simulink model "gm_Yaw"  (R2018b)
settings: Solver=ode3  StartTime=0  StopTime=TFinal  RelTol=1e-3  EnableMultiTasking=on
settings Model: Creator=The MathWorks, Inc.  LastModifiedBy=asus
settings SolverCC: MinimalZcImpactIntegration=on
settings DataIOCC: LimitDataPoints=on  SaveFormat=Array  SaveOutput=off  SaveTime=off
settings OptimizationCC: BlockReduction=off  ConditionallyExecuteInputs=off  DefaultParameterBehavior=Inlined  BufferReuse=off  PassReuseOutputArgsThreshold=0
settings DebuggingCC: AlgebraicLoopMsg=none  InheritedTsInSrcMsg=none  ParameterPrecisionLossMsg=none  ParameterTunabilityLossMsg=error  UnconnectedInputMsg=none  UnconnectedOutputMsg=none  UnconnectedLineMsg=none  BusObjectLabelMismatch=error  LibraryContextMissingDiagnostic=none  SFUnexpectedBacktrackingDiag=warning  SFNoUnconditionalDefaultTransitionDiag=warning  SFExecutionAtInitializationDiag=none
settings HardwareCC: ProdBitPerPointer=32  ProdBitPerSizeT=32  ProdBitPerPtrDiffT=32  ProdLargestAtomicInteger=Long  ProdWordSize=32  ProdHWDeviceType=ARM Compatible->ARM 9
settings ModelReferenceCC: PropagateSignalLabelsOutOfModel=off
settings SFSimCC: SimUseLocalCustomCode=off
settings RTWCC: Description=Generic Real-Time Target  GenerateReport=on  RTWUseLocalCustomCode=off  LaunchReport=on
settings CodeAppCC: ForceParamTrailComments=on  MaxIdLength=63  OperatorAnnotations=on  StateflowObjectComments=on  MATLABSourceComments=on
settings GRTTargetCC: TargetLangStandard=C89/C90 (ANSI)
settings ConfigComp: CovMetricSettings=dw  CovHtmlReporting=on  CovSaveCumulativeToWorkspaceVar=on  CovSaveSingleToWorkspaceVar=on  CovExternalEMLEnable=off  CovSFcnEnable=off

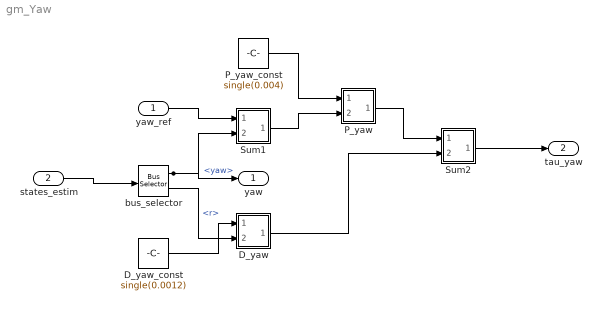
== system gm_Yaw ==
  yaw_ref : Inport  OutDataTypeStr=single  PortDimensions=1  SampleTime=0.005
  states_estim : Inport  Port=2  OutDataTypeStr=Bus: statesEstim_t  PortDimensions=1  SampleTime=0.005  BusOutputAsStruct=on
  D_yaw : Subsystem
      mask Display: disp('NFP\nmul');
  D_yaw_const : Constant  Value=single(0.0012)  OutDataTypeStr=single  SampleTime=-1
  P_yaw : Subsystem
      mask Display: disp('NFP\nmul');
  P_yaw_const : Constant  Value=single(0.004)  OutDataTypeStr=single  SampleTime=-1
  Sum1 : Subsystem
      mask Display: disp('NFP\nadd');
  Sum2 : Subsystem
      mask Display: disp('NFP\nadd');
  bus_selector : BusSelector  OutputSignals=yaw,r
  yaw : Outport  OutDataTypeStr=single  PortDimensions=1  SampleTime=[0.0050000000000000001,0]
  tau_yaw : Outport  Port=2  OutDataTypeStr=single  PortDimensions=1  SampleTime=[0.0050000000000000001,0]
  wires:
  yaw_ref/1 -> Sum1/1(In1)
  states_estim/1 -> bus_selector/1
  bus_selector/1 -> Sum1/2(In2), yaw/1  "<yaw>"
  bus_selector/2 -> D_yaw/2(In2)  "<r>"
  D_yaw_const/1 -> D_yaw/1(In1)
  P_yaw_const/1 -> P_yaw/1(In1)
  Sum1/1(Out1) -> P_yaw/2(In2)
  Sum2/1(Out1) -> tau_yaw/1
  D_yaw/1(Out1) -> Sum2/2(In2)
  P_yaw/1(Out1) -> Sum2/1(In1)

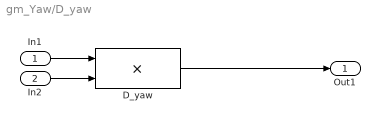
== system gm_Yaw/D_yaw ==
  In1 : Inport
  In2 : Inport  Port=2
  D_yaw : Product  Inputs=**  OutDataTypeStr=single  SampleTime=0.005
  Out1 : Outport
  wires:
  In1/1 -> D_yaw/1
  In2/1 -> D_yaw/2
  D_yaw/1 -> Out1/1

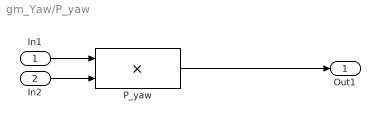
== system gm_Yaw/P_yaw ==
  In1 : Inport
  In2 : Inport  Port=2
  P_yaw : Product  Inputs=**  OutDataTypeStr=single  SampleTime=0.005
  Out1 : Outport
  wires:
  In1/1 -> P_yaw/1
  In2/1 -> P_yaw/2
  P_yaw/1 -> Out1/1

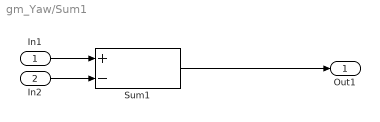
== system gm_Yaw/Sum1 ==
  In1 : Inport
  In2 : Inport  Port=2
  Sum1 : Sum  Inputs=+-  OutDataTypeStr=single  SampleTime=0.005  SaturateOnIntegerOverflow=on  InputSameDT=on
  Out1 : Outport
  wires:
  In1/1 -> Sum1/1
  In2/1 -> Sum1/2
  Sum1/1 -> Out1/1

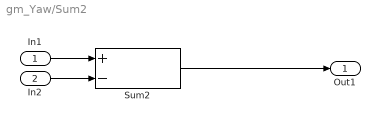
== system gm_Yaw/Sum2 ==
  In1 : Inport
  In2 : Inport  Port=2
  Sum2 : Sum  Inputs=+-  OutDataTypeStr=single  SampleTime=0.005  SaturateOnIntegerOverflow=on  InputSameDT=on
  Out1 : Outport
  wires:
  In1/1 -> Sum2/1
  In2/1 -> Sum2/2
  Sum2/1 -> Out1/1
